simulink model "pllconv"  (R2021a)
settings: Solver=ode4  StartTime=0.0  StopTime=3  RelTol=1e-3
libraries: spsVoltageMeasurementLib x7, spsACVoltageSourceLib x6, spsIGBTDiodeLib x6, spsSeriesRLCBranchLib x6, spsCurrentMeasurementLib x5, spsabctodq0Lib x3, spsGroundLib x2, simulink x1, spsdq0toabcLib x1, spspowerguiLib x1, spsDCVoltageSourceLib x1, spsThreePhaseParallelRLCLoadLib x1
settings Model: Creator=aks  LastModifiedBy=aks
settings SolverCC: ZeroCrossControl=DisableAll
settings DataIOCC: Refine=100

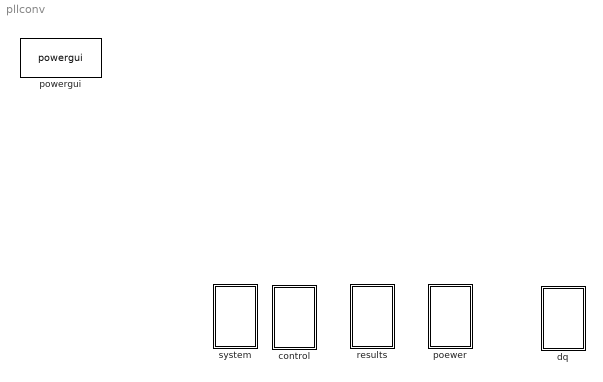
== system pllconv ==
  control : Subsystem
  dq : Subsystem
  poewer : Subsystem
  powergui : spspowerguiLib/powergui  Priority=1  SimulationMode=Discrete  SampleTime=1e-5  frequency=60  Iterations=50  frequencyindice=50  Pbase=100e6  ErrMax=1e-4  UnitsV=kV  UnitsW=MW  buscounter=0  FunctionMessages=off  echomessages=off  EnableUseOfTLC=off  CurrentSourceSwitches=off  DisableSnubberDevices=off  DisableRonSwitches=off  DisableVfSwitches=off  DisplayEquations=off  AutomaticDiscreteSolvers=off  SolverType=Tustin/Backward Euler (TBE)  Interpol=off  ExternalGateDelay=off  methode=off  Ts=100  x0status=blocks  SPID=on  SwTol=0  HookPort=off  NonlinearTolerance=1e-4  nMaxIteration=100  ContinueOnMaxIteration=off  RestoreLinks=warning  ResistiveCurrentMeasurement=off  Frange=[0:2:500]  Ylog=off  Xlog=on  ShowGrid=off  save=off  variable=ZData  structure=0  ZoomFFT=off  StartTime=0.0  cycles=1  DisplayStyle=1  fundamental=60  FreqAxis=off  MaxFrequency=1000  frequencyindicesteady=1  RmsSteady=1  display=off
  results : Subsystem
  system : Subsystem

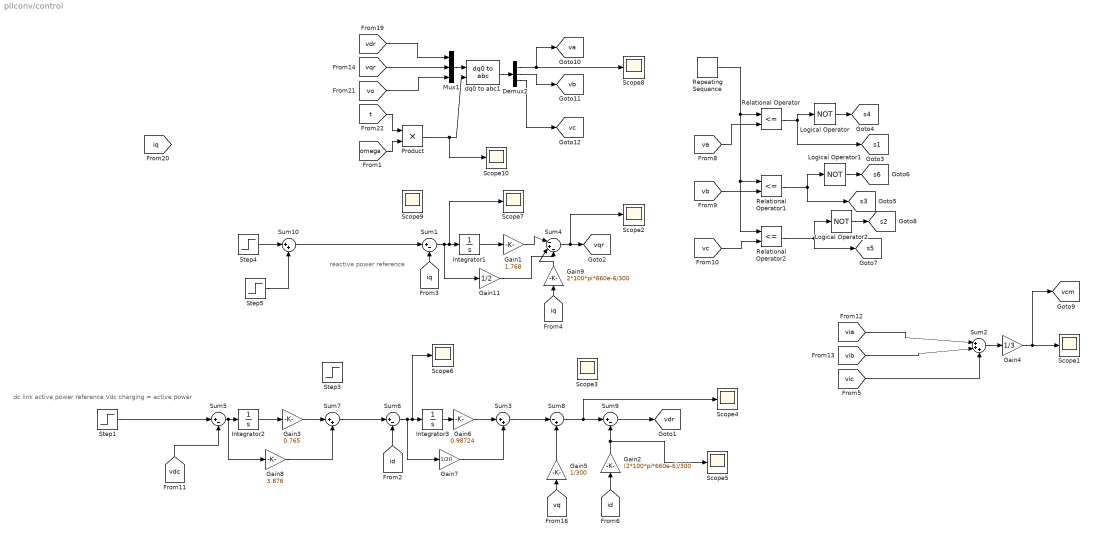
== system pllconv/control ==
  note: dc link active power reference Vdc charging = active power
  note: reactive power reference
  Demux2 : Demux  Outputs=3
  Gain1 : Gain  Gain=1.768
  Gain11 : Gain  Gain=1/2
  Gain2 : Gain  Gain=(2*100*pi*660e-6)/300
  Gain3 : Gain  Gain=0.765
  Gain4 : Gain  Gain=1/3
  Gain5 : Gain  Gain=1/300
  Gain6 : Gain  Gain=0.98724
  Gain7 : Gain  Gain=1/20
  Gain8 : Gain  Gain=3.876
  Gain9 : Gain  Gain=2*100*pi*660e-6/300
  Integrator1 : Integrator
  Integrator2 : Integrator
  Integrator3 : Integrator
  Logical Operator : Logic  Operator=NOT  AllPortsSameDT=off  OutDataTypeStr=boolean
  Logical Operator1 : Logic  Operator=NOT  AllPortsSameDT=off  OutDataTypeStr=boolean
  Logical Operator2 : Logic  Operator=NOT  AllPortsSameDT=off  OutDataTypeStr=boolean
  Mux1 : Mux  Inputs=3
  Product : Product
  Relational Operator : RelationalOperator  Operator=<=  OutDataTypeStr=boolean  RndMeth=Simplest
  Relational Operator1 : RelationalOperator  Operator=<=  OutDataTypeStr=boolean  RndMeth=Simplest
  Relational Operator2 : RelationalOperator  Operator=<=  OutDataTypeStr=boolean  RndMeth=Simplest
  Repeating Sequence : simulink/Sources/Repeating Sequence  rep_seq_t=[0 (1/20000) (1/10000) (3/20000) (1/5000)]  rep_seq_y=[0 1 0 -1 0]
  Scope{1..10} (10 alike) : Scope
  Step1 : Step  Time=1.5  Before=1000  After=500  SampleTime=0
  Step3 : Step  Before=10  After=-10  SampleTime=0
  Step4 : Step  Time=0.5  Before=1000  After=0  SampleTime=0
  Step5 : Step  Time=2.5  After=-1000  SampleTime=0
  Sum{1,5..6,9} (4 alike) : Sum  Inputs=|+-
  Sum10 : Sum  Inputs=|++
  Sum2 : Sum  Inputs=|+++
  Sum3 : Sum  Inputs=|++
  Sum4 : Sum  Inputs=|-+-
  Sum7 : Sum  Inputs=|++
  Sum8 : Sum  Inputs=|-+
  dq0 to abc1 : spsdq0toabcLib/dq0 to abc  Alignment=90 degrees behind phase A axis
  tag scope: s1=global, s2=global, s3=global, s4=global, s5=global, s6=global, va=global, vb=global, vc=global, vcm=global, vdr=global, vqr=global
  wires:
  Sum1/1 -> Gain11/1, Scope7/1, Integrator1/1
  Integrator1/1 -> Gain1/1
  Gain1/1 -> Sum4/1
  Repeating Sequence/1 -> Relational Operator2/1, Relational Operator1/1, Relational Operator/1
  Relational Operator/1 -> [s1], Logical Operator/1
  Logical Operator/1 -> [s4]
  Logical Operator1/1 -> [s6]
  Relational Operator1/1 -> Logical Operator1/1, [s3]
  Relational Operator2/1 -> Logical Operator2/1, [s5]
  Logical Operator2/1 -> [s2]
  [vdc] -> Sum5/2
  [id] -> Gain2/1
  [iq] -> Gain9/1
  Gain9/1 -> Sum4/2
  Sum6/1 -> Gain7/1, Scope6/1, Integrator3/1
  Integrator3/1 -> Gain6/1
  Sum8/1 -> Scope4/1, Sum9/1
  Gain2/1 -> Scope5/1, Sum9/2
  Gain5/1 -> Sum8/2
  Sum5/1 -> Gain8/1, Integrator2/1
  Integrator2/1 -> Gain3/1
  [vic] -> Sum2/3
  [vib] -> Sum2/2
  [via] -> Sum2/1
  Sum2/1 -> Gain4/1
  Gain4/1 -> [vcm], Scope1/1
  [t] -> Product/1
  dq0 to abc1/1 -> Demux2/1
  Product/1 -> Scope10/1, dq0 to abc1/2
  [vo] -> Mux1/3
  Mux1/1 -> dq0 to abc1/1
  Demux2/1 -> Scope8/1, [va]
  Demux2/2 -> [vb]
  Demux2/3 -> [vc]
  [va] -> Relational Operator/2
  [vb] -> Relational Operator1/2
  [vc] -> Relational Operator2/2
  [vq] -> Gain5/1
  [vdr] -> Mux1/1
  [vqr] -> Mux1/2
  Sum9/1 -> [vdr]
  Sum4/1 -> Scope2/1, [vqr]
  Gain7/1 -> Sum3/2
  Gain6/1 -> Sum3/1
  Sum3/1 -> Sum8/1
  [iq] -> Sum1/2
  [id] -> Sum6/2
  Gain3/1 -> Sum7/1
  Gain8/1 -> Sum7/2
  Gain11/1 -> Sum4/3
  [omega] -> Product/2
  Step1/1 -> Sum5/1
  Sum10/1 -> Sum1/1
  Sum7/1 -> Sum6/1
  Step4/1 -> Sum10/1
  Step5/1 -> Sum10/2

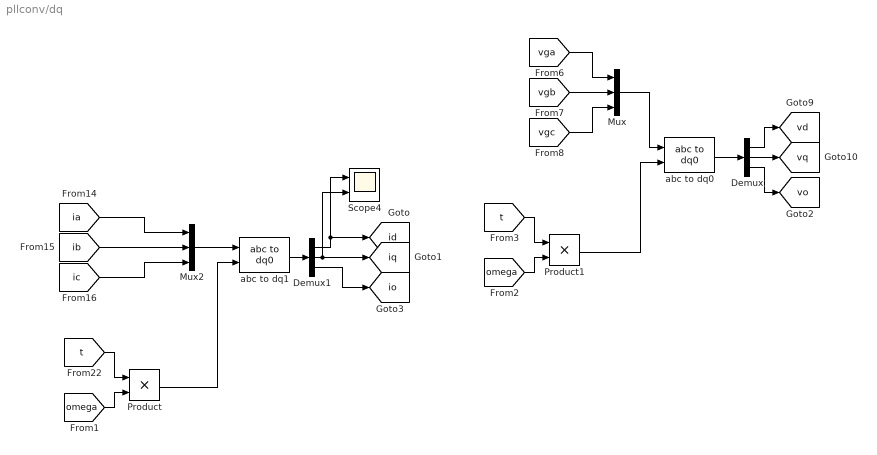
== system pllconv/dq ==
  Demux : Demux  Outputs=3
  Demux1 : Demux  Outputs=3
  Mux : Mux  Inputs=3
  Mux2 : Mux  Inputs=3
  Product : Product
  Product1 : Product
  Scope4 : Scope  NumInputPorts=2
  abc to dq0 : spsabctodq0Lib/abc to dq0  Alignment=90 degrees behind phase A axis
  abc to dq1 : spsabctodq0Lib/abc to dq0  Alignment=90 degrees behind phase A axis
  tag scope: id=global, io=global, iq=global, vd=global, vo=global, vq=global
  wires:
  Demux/2 -> [vq]
  Demux/1 -> [vd]
  [vgb] -> Mux/2
  [vga] -> Mux/1
  [vgc] -> Mux/3
  Mux/1 -> abc to dq0/1
  abc to dq0/1 -> Demux/1
  Demux/3 -> [vo]
  Mux2/1 -> abc to dq1/1
  [ia] -> Mux2/1
  [ic] -> Mux2/3
  [ib] -> Mux2/2
  abc to dq1/1 -> Demux1/1
  Demux1/1 -> Scope4/1, [id]
  Demux1/2 -> [iq], Scope4/2
  Demux1/3 -> [io]
  [t] -> Product/1
  Product/1 -> abc to dq1/2
  [omega] -> Product/2
  [t] -> Product1/1
  Product1/1 -> abc to dq0/2
  [omega] -> Product1/2

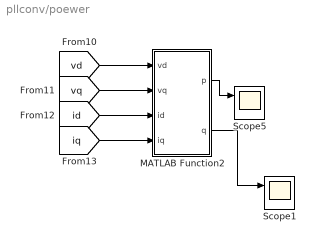
== system pllconv/poewer ==
  MATLAB Function2 : MATLAB Function  TreatAsAtomicUnit=on
  Scope1 : Scope  NumInputPorts=2
  Scope5 : Scope  NumInputPorts=2
  wires:
  [vq] -> MATLAB Function2/2(vq)
  [iq] -> MATLAB Function2/4(iq)
  [vd] -> MATLAB Function2/1(vd)
  MATLAB Function2/1(p) -> Scope5/1
  [id] -> MATLAB Function2/3(id)
  MATLAB Function2/2(q) -> Scope1/1

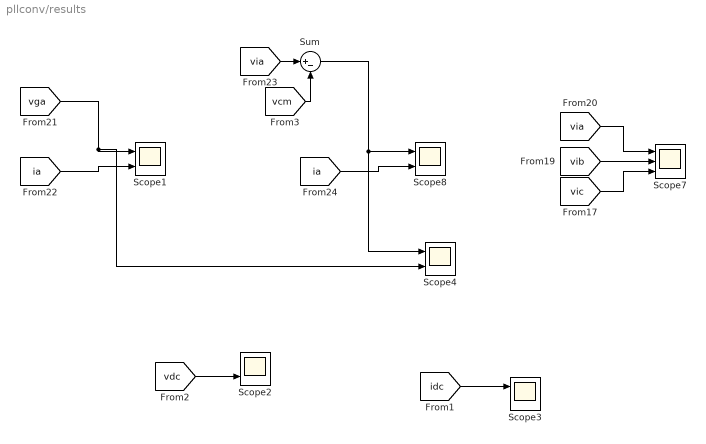
== system pllconv/results ==
  Scope{1..4,8} (5 alike) : Scope  NumInputPorts=2
  Scope7 : Scope  NumInputPorts=3
  Sum : Sum  Inputs=|+-
  wires:
  [vga] -> Scope4/2, Scope1/1
  [ia] -> Scope8/2
  [vic] -> Scope7/3
  [ia] -> Scope1/2
  [vib] -> Scope7/2
  [via] -> Scope7/1
  [vdc] -> Scope2/2
  [idc] -> Scope3/1
  [via] -> Sum/1
  [vcm] -> Sum/2
  Sum/1 -> Scope4/1, Scope8/1

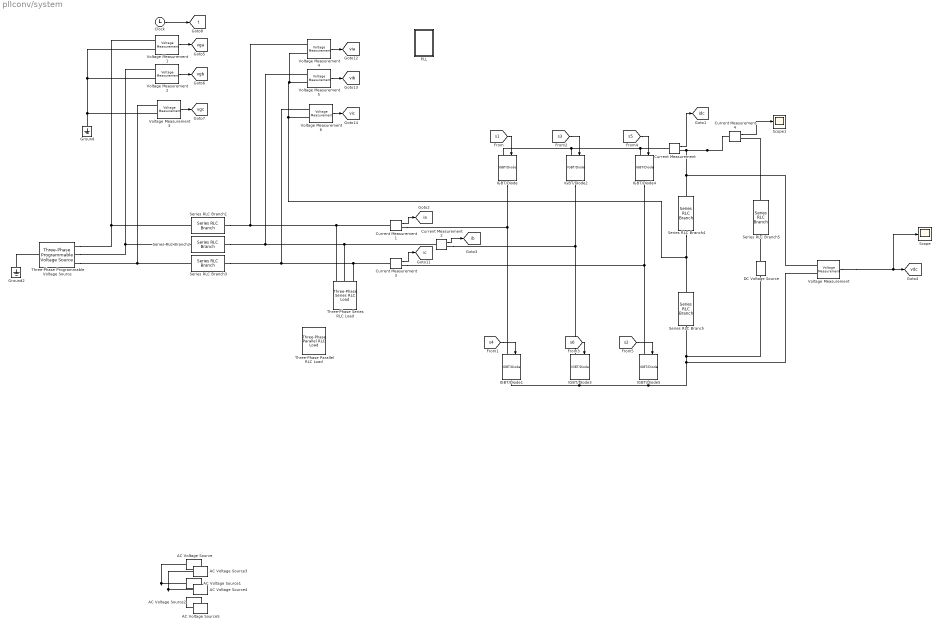
== system pllconv/system ==
  AC Voltage Source : spsACVoltageSourceLib/AC Voltage Source  Amplitude=168*sqrt(2)  Phase=0  Frequency=50  SampleTime=0  Measurements=None  BusType=swing  Pref=10e3  Qref=0  Qmin=-inf  Qmax=+inf
  AC Voltage Source1 : spsACVoltageSourceLib/AC Voltage Source  Amplitude=168*sqrt(2)  Phase=-120  Frequency=50  SampleTime=0  Measurements=None  BusType=swing  Pref=10e3  Qref=0  Qmin=-inf  Qmax=+inf
  AC Voltage Source2 : spsACVoltageSourceLib/AC Voltage Source  Amplitude=168*sqrt(2)  Phase=120  Frequency=50  SampleTime=0  Measurements=None  BusType=swing  Pref=10e3  Qref=0  Qmin=-inf  Qmax=+inf
  AC Voltage Source3 : spsACVoltageSourceLib/AC Voltage Source  Amplitude=168*sqrt(2)  Phase=0  Frequency=50  SampleTime=0  Measurements=None  BusType=swing  Pref=10e3  Qref=0  Qmin=-inf  Qmax=+inf
  AC Voltage Source4 : spsACVoltageSourceLib/AC Voltage Source  Amplitude=168*sqrt(2)  Phase=-120  Frequency=50  SampleTime=0  Measurements=None  BusType=swing  Pref=10e3  Qref=0  Qmin=-inf  Qmax=+inf
  AC Voltage Source5 : spsACVoltageSourceLib/AC Voltage Source  Amplitude=168*sqrt(2)  Phase=120  Frequency=50  SampleTime=0  Measurements=None  BusType=swing  Pref=10e3  Qref=0  Qmin=-inf  Qmax=+inf
  Clock : Clock
  Current Measurement{,1..4} (5 alike) : spsCurrentMeasurementLib/Current Measurement  PhasorSimulation=off  OutputType=Complex  PSBequivalent=0
  DC Voltage Source : spsDCVoltageSourceLib/DC Voltage Source  Amplitude=800  Measurements=None
  Ground : spsGroundLib/Ground  LConnTagsString=a
  Ground2 : spsGroundLib/Ground  LConnTagsString=a
  IGBT/Diode{,1..5} (6 alike) : spsIGBTDiodeLib/IGBT//Diode  Ron=1e-3  Rs=1e5  Cs=inf  Measurements=off
  PLL : Subsystem
  Scope : Scope
  Scope1 : Scope
  Series RLC Branch : spsSeriesRLCBranchLib/Series RLC Branch  LConnTagsString=__new0  RConnTagsString=__new0  BranchType=C  Resistance=10000  Inductance=1e-3  SetiL0=off  InitialCurrent=0  Capacitance=2*(6750e-6)  Setx0=on  InitialVoltage=0  Measurements=None
  Series RLC Branch1 : spsSeriesRLCBranchLib/Series RLC Branch  LConnTagsString=__new0  RConnTagsString=__new0  BranchType=RL  Resistance=2e-3  Inductance=660e-6  SetiL0=off  InitialCurrent=0  Capacitance=1e-6  Setx0=off  InitialVoltage=0  Measurements=None
  Series RLC Branch2 : spsSeriesRLCBranchLib/Series RLC Branch  LConnTagsString=__new0  RConnTagsString=__new0  BranchType=RL  Resistance=2e-3  Inductance=660e-6  SetiL0=off  InitialCurrent=0  Capacitance=1e-6  Setx0=off  InitialVoltage=0  Measurements=None
  Series RLC Branch3 : spsSeriesRLCBranchLib/Series RLC Branch  LConnTagsString=__new0  RConnTagsString=__new0  BranchType=RL  Resistance=2e-3  Inductance=660e-6  SetiL0=off  InitialCurrent=0  Capacitance=1e-6  Setx0=off  InitialVoltage=0  Measurements=None
  Series RLC Branch4 : spsSeriesRLCBranchLib/Series RLC Branch  LConnTagsString=__new0  RConnTagsString=__new0  BranchType=C  Resistance=10000  Inductance=1e-3  SetiL0=off  InitialCurrent=0  Capacitance=2*(6750e-6)  Setx0=on  InitialVoltage=0  Measurements=None
  Series RLC Branch5 : spsSeriesRLCBranchLib/Series RLC Branch  LConnTagsString=__new0  RConnTagsString=__new0  BranchType=R  Resistance=10  Inductance=100  SetiL0=off  InitialCurrent=0  Capacitance=1e-6  Setx0=off  InitialVoltage=0  Measurements=None
  Three-Phase Parallel RLC Load : spsThreePhaseParallelRLCLoadLib/Three-Phase Parallel RLC Load  LConnTagsString=A|B|C  Configuration=Y (grounded)  NominalVoltage=1000  Vabc=[1e3 1e3 1e3]  Vabcp=[1e3 1e3 1e3]  NominalFrequency=50  UnbalancedPower=off  ActivePower=0  InductivePower=0  CapacitivePower=600  Pabc=[10e3 9e3 11e3]  QLabc=[100 90 110]  QCabc=[100 90 110]  Pabcp=[10e3 9e3 11e3]  QLabcp=[100 90 110]  QCabcp=[100 90 110]  Measurements=None  LoadType=constant Z
  Three-Phase Programmable Voltage Source : spsThreePhaseProgrammableVoltageSourceLib/Three-Phase Programmable Voltage Source  PositiveSequence="[168*sqrt(3)  0 50]"  VariationEntity=None  VariationType=Table of time-amplitude pairs  VariationTypeAlt=Step  VariationStep=0.25  VariationRate=10  VariationMagnitude=0.3  VariationFrequency=2  VariationTiming=[0.5 1]  VariationPhaseA=off  Amplitudes=[1 0.8 1.2 1.0]  TimeValues=[0 0.1 0.15 0.2]  HarmonicGeneration=off  HarmonicA=[3 0.2 -25 0]  HarmonicB=[2 0.15 35 2]  Timing="[0.05  3]"  BusType=swing  Pref=0  Qref=0  Qmin=-inf  Qmax=inf
  Three-Phase Series RLC Load : spsThreePhaseSeriesRLCLoadLib/Three-Phase Series RLC Load  LConnTagsString=A|B|C  Configuration=Y (grounded)  NominalVoltage=1000  Vabc=[1e3 1e3 1e3]  Vabcp=[1e3 1e3 1e3]  NominalFrequency=50  UnbalancedPower=off  ActivePower=10e3  InductivePower=100  CapacitivePower=0  Pabc=[10e3 9e3 11e3]  QLabc=[100 90 110]  QCabc=[100 90 110]  Pabcp=[10e3 9e3 11e3]  QLabcp=[100 90 110]  QCabcp=[100 90 110]  Measurements=None  LoadType=constant Z
  Voltage Measurement{,1..6} (7 alike) : spsVoltageMeasurementLib/Voltage Measurement  PhasorSimulation=off  OutputType=Complex  PSBequivalent=0
  tag scope: ia=global, ib=global, ic=global, idc=global, t=global, vdc=global, vga=global, vgb=global, vgc=global, via=global, vib=global, vic=global
  wires:
  Current Measurement2/1 -> [ib]
  Voltage Measurement2/1 -> [vgb]
  Voltage Measurement3/1 -> [vgc]
  Voltage Measurement/1 -> [vdc], Scope/1
  Clock/1 -> [t]
  Voltage Measurement5/1 -> [vib]
  Current Measurement3/1 -> [ic]
  Voltage Measurement4/1 -> [via]
  Voltage Measurement6/1 -> [vic]
  Current Measurement/1 -> [idc]
  Current Measurement1/1 -> [ia]
  Voltage Measurement1/1 -> [vga]
  [s1] -> IGBT/Diode/1
  [s3] -> IGBT/Diode2/1
  [s5] -> IGBT/Diode4/1
  [s2] -> IGBT/Diode5/1
  [s6] -> IGBT/Diode3/1
  [s4] -> IGBT/Diode1/1
  Current Measurement4/1 -> Scope1/1
  connections:
  IGBT/Diode/RConn1 -- Current Measurement1/RConn1 -- IGBT/Diode1/LConn1
  IGBT/Diode/LConn1 -- Current Measurement/LConn1 -- IGBT/Diode4/LConn1 -- IGBT/Diode2/LConn1
  Series RLC Branch2/RConn1 -- Voltage Measurement5/LConn1 -- Current Measurement2/LConn1 -- Three-Phase Series RLC Load/LConn2
  Series RLC Branch3/RConn1 -- Voltage Measurement6/LConn1 -- Three-Phase Series RLC Load/LConn3 -- Current Measurement3/LConn1
  IGBT/Diode1/RConn1 -- IGBT/Diode3/RConn1 -- Voltage Measurement/LConn2 -- DC Voltage Source/LConn1 -- Series RLC Branch/RConn1 -- IGBT/Diode5/RConn1
  Series RLC Branch1/RConn1 -- Voltage Measurement4/LConn1 -- Three-Phase Series RLC Load/LConn1 -- Current Measurement1/LConn1
  IGBT/Diode4/RConn1 -- IGBT/Diode5/LConn1 -- Current Measurement3/RConn1
  Voltage Measurement1/LConn1 -- Three-Phase Programmable Voltage Source/RConn1 -- Series RLC Branch1/LConn1
  Voltage Measurement2/LConn1 -- Three-Phase Programmable Voltage Source/RConn2 -- Series RLC Branch2/LConn1
  IGBT/Diode2/RConn1 -- Current Measurement2/RConn1 -- IGBT/Diode3/LConn1
  Ground/LConn1 -- Voltage Measurement1/LConn2 -- Voltage Measurement2/LConn2 -- Voltage Measurement3/LConn2
  Voltage Measurement3/LConn1 -- Three-Phase Programmable Voltage Source/RConn3 -- Series RLC Branch3/LConn1
  Voltage Measurement4/LConn2 -- Series RLC Branch/LConn1 -- Series RLC Branch4/RConn1 -- Voltage Measurement6/LConn2 -- Voltage Measurement5/LConn2
  Series RLC Branch5/RConn1 -- Current Measurement4/RConn1
  Ground2/LConn1 -- Three-Phase Programmable Voltage Source/LConn1
  AC Voltage Source1/LConn1 -- AC Voltage Source/LConn1
  AC Voltage Source4/LConn1 -- AC Voltage Source3/LConn1
  DC Voltage Source/RConn1 -- Series RLC Branch5/LConn1
  Voltage Measurement/LConn1 -- Series RLC Branch4/LConn1 -- Current Measurement/RConn1 -- Current Measurement4/LConn1

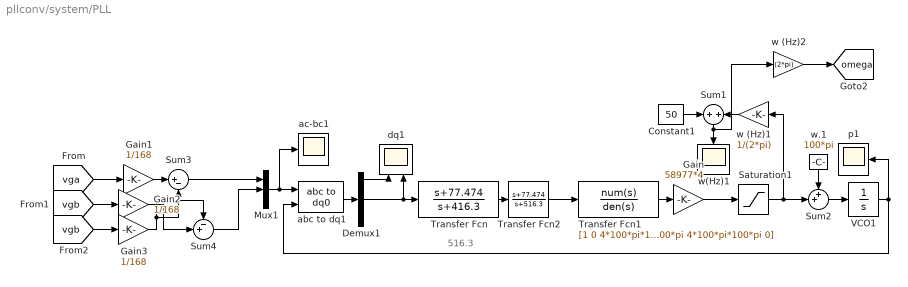
== system pllconv/system/PLL ==
  note: 516.3
  Constant1 : Constant  Value=50
  Demux1 : Demux  Outputs=3
  Gain : Gain  Gain=58977*4
  Gain1 : Gain  Gain=1/168
  Gain2 : Gain  Gain=1/168
  Gain3 : Gain  Gain=1/168
  Mux1 : Mux  Inputs=3
  Saturation1 : Saturate  UpperLimit=500  LowerLimit=-500
  Sum1 : Sum  Inputs=+|+
  Sum2 : Sum  Inputs=++|
  Sum3 : Sum  Inputs=|+-
  Sum4 : Sum  Inputs=-+|
  Transfer Fcn : TransferFcn  Numerator=[1 77.474]  Denominator=[1 416.3]
  Transfer Fcn1 : TransferFcn  Numerator=[1 0 4*100*pi*100*pi]  Denominator=[1 4*100*pi 4*100*pi*100*pi 0]
  Transfer Fcn2 : TransferFcn  Numerator=[1 77.474]  Denominator=[1 516.3]
  VCO1 : Integrator  UpperSaturationLimit=2*pi  LowerSaturationLimit=0  WrapState=on  WrappedStateUpperValue=2*pi  WrappedStateLowerValue=0
  abc to dq1 : spsabctodq0Lib/abc to dq0  Alignment=90 degrees behind phase A axis
  ac-bc1 : Scope
  dq1 : Scope  NumInputPorts=2
  p1 : Scope
  w (Hz)1 : Gain  Gain=1/(2*pi)
  w (Hz)2 : Gain  Gain=(2*pi)
  w(Hz)1 : Scope
  w.1 : Constant  Value=100*pi
  tag scope: omega=global
  wires:
  w (Hz)1/1 -> Sum1/2
  abc to dq1/1 -> Demux1/1
  Sum3/1 -> Mux1/1
  Constant1/1 -> Sum1/1
  [vga] -> Gain1/1
  Transfer Fcn/1 -> Transfer Fcn2/1
  w.1/1 -> Sum2/1
  Transfer Fcn2/1 -> Transfer Fcn1/1
  Sum2/1 -> VCO1/1
  Demux1/2 -> Transfer Fcn/1, dq1/2
  VCO1/1 -> abc to dq1/2, p1/1
  Sum1/1 -> w (Hz)2/1, w(Hz)1/1
  Transfer Fcn1/1 -> Gain/1
  Sum4/1 -> Mux1/2
  Demux1/1 -> dq1/1
  Saturation1/1 -> Sum2/2, w (Hz)1/1
  Gain/1 -> Saturation1/1
  Mux1/1 -> ac-bc1/1, abc to dq1/1
  Gain1/1 -> Sum3/1
  [vgb] -> Gain2/1
  Gain2/1 -> Sum4/2
  [vgb] -> Gain3/1
  Gain3/1 -> Sum3/2, Sum4/1
  w (Hz)2/1 -> [omega]

== matlab function pllconv/poewer/MATLAB Function2 ==
  data: vd input; p output; vq input; id input; iq input; q output
function [p,q]= fcn(vd,vq,id,iq)
p= (vd*id+vq*iq);
q=(vd*iq-vq*id);
